simulink model "MyProjectPicture"  (R2019a)
settings: Solver=VariableStepAuto  StartTime=0.0  StopTime=10.0  RelTol=1e-3
values from neighbouring files (symbols this model uses):
  R1 = 2    [MyProjectScript.m]
  R2 = 1.5    [MyProjectScript.m]
  Rh_cons = Rh(a)    [MyProjectScript.m]
  Rh_par = Rh(a)    [MyProjectScript.m]
libraries: fl_lib x20, nesl_utility x12
settings Model: Creator=Алена  LastModifiedBy=Алена
settings DataIOCC: ReturnWorkspaceOutputs=off

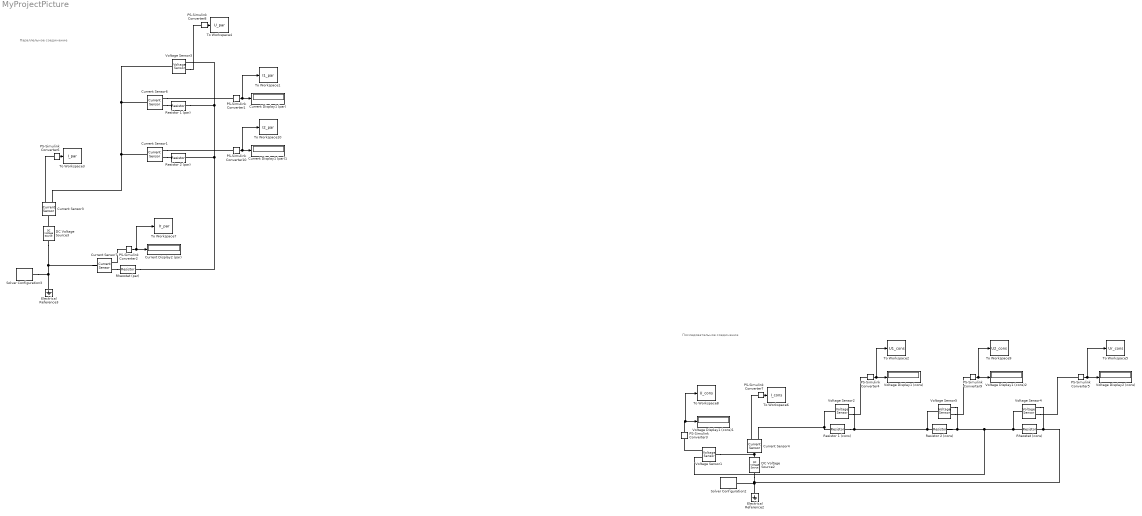
== system MyProjectPicture ==
  note: Параллельное соединение
  note: Последовательное соединение
  Current Display1 (par) : Display
  Current Display1 (par)1 : Display
  Current Display2 (par) : Display
  Current Sensor{1,3..4,6..7} (5 alike) : fl_lib/Electrical/Electrical Sensors/Current Sensor
  DC Voltage Source2 : fl_lib/Electrical/Electrical Sources/DC Voltage Source  v0=Uist_cons V
  DC Voltage Source3 : fl_lib/Electrical/Electrical Sources/DC Voltage Source  v0=Uist_par V
  Electrical Reference2 : fl_lib/Electrical/Electrical Elements/Electrical Reference
  Electrical Reference3 : fl_lib/Electrical/Electrical Elements/Electrical Reference
  PS-Simulink Converter{1..10} (10 alike) : nesl_utility/PS-Simulink Converter  PhysicalDomain=network_engine_domain  SubClassName=ps_output  LeftPortType=input  RightPortType=output  PseudoPeriodic=off  Frequencies=[]  Unit=1  AffineConversion=off
  Resistor 1 (cons) : fl_lib/Electrical/Electrical Elements/Resistor  R=R1 Ohm  i_specify=off  i_priority=None  i=0 A  i_nominal_specify=off  i_nominal_unit=A  i_nominal_value=1  v_specify=off  v_priority=None  v=0 V  v_nominal_specify=off  v_nominal_unit=V  v_nominal_value=1
  Resistor 1 (par) : fl_lib/Electrical/Electrical Elements/Resistor  R=R1 Ohm  i_specify=off  i_priority=None  i=0 A  i_nominal_specify=off  i_nominal_unit=A  i_nominal_value=1  v_specify=off  v_priority=None  v=0 V  v_nominal_specify=off  v_nominal_unit=V  v_nominal_value=1
  Resistor 2 (cons) : fl_lib/Electrical/Electrical Elements/Resistor  R=R2 Ohm  i_specify=off  i_priority=None  i=0 A  i_nominal_specify=off  i_nominal_unit=A  i_nominal_value=1  v_specify=off  v_priority=None  v=0 V  v_nominal_specify=off  v_nominal_unit=V  v_nominal_value=1
  Resistor 2 (par) : fl_lib/Electrical/Electrical Elements/Resistor  R=R2 Ohm  i_specify=off  i_priority=None  i=0 A  i_nominal_specify=off  i_nominal_unit=A  i_nominal_value=1  v_specify=off  v_priority=None  v=0 V  v_nominal_specify=off  v_nominal_unit=V  v_nominal_value=1
  Rheostat (cons) : fl_lib/Electrical/Electrical Elements/Resistor  R=Rh_cons Ohm  i_specify=off  i_priority=None  i=0 A  i_nominal_specify=off  i_nominal_unit=A  i_nominal_value=1  v_specify=off  v_priority=None  v=0 V  v_nominal_specify=off  v_nominal_unit=V  v_nominal_value=1
  Rheostat (par) : fl_lib/Electrical/Electrical Elements/Resistor  R=Rh_par Ohm  i_specify=off  i_priority=None  i=0 A  i_nominal_specify=off  i_nominal_unit=A  i_nominal_value=1  v_specify=off  v_priority=None  v=0 V  v_nominal_specify=off  v_nominal_unit=V  v_nominal_value=1
  Solver Configuration2 : nesl_utility/Solver Configuration  PhysicalDomain=network_engine_domain  SubClassName=solver  LeftPortType=input  RightPortType=generic  Tones=[]  Harmonics=[]  SimulateNoise=off  Profile=off  UseLocalSampling=off  EnableSwitchedLinearOptims=on  FrequencyDomain=off  UseCCode=off  RelTol=0.001  AbsTol=1e-06  MinStep=1e-09  ToWorkspace=off  RevertToSquareIcSolve=off  NumHomotopyIterations=100  PhasorMode=off  PhasorModeNumHarmonics=1  DoDC=off  ResidualTolerance=1e-09  UseLocalSolver=off  LocalSolverChoice=NE_BACKWARD_EULER_ADVANCER  LocalSolverSampleTime=0.001  DoFixedCost=off  MaxNonlinIter=3  MaxModeIter=2  LinearAlgebra=auto  EquationFormulation=NE_TIME_EF  DelaysMemoryBudget=1024  AutomaticFiltering=on  FilteringTimeConstant=0.001  PartitionStorageMethod=AS_NEEDED  PartitionMemoryBudget=1024  PartitionMethod=ROBUST
  Solver Configuration3 : nesl_utility/Solver Configuration  PhysicalDomain=network_engine_domain  SubClassName=solver  LeftPortType=input  RightPortType=generic  Tones=[]  Harmonics=[]  SimulateNoise=off  Profile=off  UseLocalSampling=off  EnableSwitchedLinearOptims=on  FrequencyDomain=off  UseCCode=off  RelTol=0.001  AbsTol=1e-06  MinStep=1e-09  ToWorkspace=off  RevertToSquareIcSolve=off  NumHomotopyIterations=100  PhasorMode=off  PhasorModeNumHarmonics=1  DoDC=off  ResidualTolerance=1e-09  UseLocalSolver=off  LocalSolverChoice=NE_BACKWARD_EULER_ADVANCER  LocalSolverSampleTime=0.001  DoFixedCost=off  MaxNonlinIter=3  MaxModeIter=2  LinearAlgebra=auto  EquationFormulation=NE_TIME_EF  DelaysMemoryBudget=1024  AutomaticFiltering=on  FilteringTimeConstant=0.001  PartitionStorageMethod=AS_NEEDED  PartitionMemoryBudget=1024  PartitionMethod=ROBUST
  To Workspace1 : ToWorkspace  VariableName=I1_par  SaveFormat=Structure  SampleTime=-1
      settings: Save2DSignal=2-D array (concatenate along first dimension)
  To Workspace10 : ToWorkspace  VariableName=I2_par  SaveFormat=Structure  SampleTime=-1
      settings: Save2DSignal=2-D array (concatenate along first dimension)
  To Workspace2 : ToWorkspace  VariableName=U1_cons  SaveFormat=Structure  SampleTime=-1
      settings: Save2DSignal=2-D array (concatenate along first dimension)
  To Workspace3 : ToWorkspace  VariableName=I_par  SaveFormat=Structure  SampleTime=-1
      settings: Save2DSignal=2-D array (concatenate along first dimension)
  To Workspace4 : ToWorkspace  VariableName=U_par  SaveFormat=Structure  SampleTime=-1
      settings: Save2DSignal=2-D array (concatenate along first dimension)
  To Workspace5 : ToWorkspace  VariableName=Ur_cons  SaveFormat=Structure  SampleTime=-1
      settings: Save2DSignal=2-D array (concatenate along first dimension)
  To Workspace6 : ToWorkspace  VariableName=I_cons  SaveFormat=Structure  SampleTime=-1
      settings: Save2DSignal=2-D array (concatenate along first dimension)
  To Workspace7 : ToWorkspace  VariableName=Ir_par  SaveFormat=Structure  SampleTime=-1
      settings: Save2DSignal=2-D array (concatenate along first dimension)
  To Workspace8 : ToWorkspace  VariableName=U_cons  SaveFormat=Structure  SampleTime=-1
      settings: Save2DSignal=2-D array (concatenate along first dimension)
  To Workspace9 : ToWorkspace  VariableName=U2_cons  SaveFormat=Structure  SampleTime=-1
      settings: Save2DSignal=2-D array (concatenate along first dimension)
  Voltage Display1 (cons) : Display
  Voltage Display1 (cons)1 : Display
  Voltage Display1 (cons)2 : Display
  Voltage Display2 (cons) : Display
  Voltage Sensor{1..5} (5 alike) : fl_lib/Electrical/Electrical Sensors/Voltage Sensor
  wires:
  PS-Simulink Converter4/1 -> To Workspace2/1, Voltage Display1 (cons)/1
  PS-Simulink Converter5/1 -> To Workspace5/1, Voltage Display2 (cons)/1
  PS-Simulink Converter7/1 -> To Workspace6/1
  PS-Simulink Converter6/1 -> To Workspace3/1
  PS-Simulink Converter2/1 -> To Workspace7/1, Current Display2 (par)/1
  PS-Simulink Converter8/1 -> To Workspace4/1
  PS-Simulink Converter1/1 -> To Workspace1/1, Current Display1 (par)/1
  PS-Simulink Converter3/1 -> Voltage Display1 (cons)1/1, To Workspace8/1
  PS-Simulink Converter9/1 -> To Workspace9/1, Voltage Display1 (cons)2/1
  PS-Simulink Converter10/1 -> To Workspace10/1, Current Display1 (par)1/1
  connections:
  DC Voltage Source2/RConn1 -- Voltage Sensor4/RConn2 -- Rheostat (cons)/RConn1 -- Electrical Reference2/LConn1 -- Solver Configuration2/RConn1
  DC Voltage Source2/LConn1 -- Current Sensor4/LConn1 -- Voltage Sensor1/LConn1
  Voltage Sensor2/LConn1 -- Current Sensor4/RConn2 -- Resistor 1 (cons)/LConn1
  Voltage Sensor4/LConn1 -- Voltage Sensor1/RConn2 -- Voltage Sensor5/RConn2 -- Resistor 2 (cons)/RConn1 -- Rheostat (cons)/LConn1
  Voltage Sensor2/RConn1 -- PS-Simulink Converter4/LConn1
  Voltage Sensor4/RConn1 -- PS-Simulink Converter5/LConn1
  Current Sensor4/RConn1 -- PS-Simulink Converter7/LConn1
  Voltage Sensor3/LConn1 -- Current Sensor3/RConn2 -- Current Sensor1/LConn1 -- Current Sensor6/LConn1
  Voltage Sensor3/RConn2 -- Rheostat (par)/RConn1 -- Resistor 2 (par)/RConn1 -- Resistor 1 (par)/RConn1
  Current Sensor6/RConn2 -- Resistor 1 (par)/LConn1
  Voltage Sensor3/RConn1 -- PS-Simulink Converter8/LConn1
  Current Sensor6/RConn1 -- PS-Simulink Converter1/LConn1
  DC Voltage Source3/LConn1 -- Current Sensor3/LConn1
  Current Sensor7/RConn2 -- Rheostat (par)/LConn1
  Current Sensor3/RConn1 -- PS-Simulink Converter6/LConn1
  DC Voltage Source3/RConn1 -- Current Sensor7/LConn1 -- Solver Configuration3/RConn1 -- Electrical Reference3/LConn1
  Current Sensor7/RConn1 -- PS-Simulink Converter2/LConn1
  Voltage Sensor1/RConn1 -- PS-Simulink Converter3/LConn1
  Voltage Sensor5/LConn1 -- Voltage Sensor2/RConn2 -- Resistor 1 (cons)/RConn1 -- Resistor 2 (cons)/LConn1
  Voltage Sensor5/RConn1 -- PS-Simulink Converter9/LConn1
  Current Sensor1/RConn1 -- PS-Simulink Converter10/LConn1
  Current Sensor1/RConn2 -- Resistor 2 (par)/LConn1
